simulink model "ADPSE1LEMK"  (R2018b)
settings: Solver=ode1  StartTime=0.0  StopTime=100  FixedStep=1/1000  RelTol=1e-3  AbsTol=1e-3  EnableMultiTasking=on
PostLoadFcn:
  | f_Simulink_figureplace
InitFcn:
  | ADPSE1LEMK_PreSim
values from neighbouring files (symbols this model uses):
  beta = 3    [ADPSE1LEMK_PreSim.m]
  etaa1 = 10    [ADPSE1LEMK_PreSim.m]
  etaa2 = 0.1    [ADPSE1LEMK_PreSim.m]
  etac1 = 1    [ADPSE1LEMK_PreSim.m]
  etac2 = 2    [ADPSE1LEMK_PreSim.m]
  Gamma0 = 100*eye(L)    [ADPSE1LEMK_PreSim.m]
  GammaBar = 100000    [ADPSE1LEMK_PreSim.m]
  GG = [GG;phi_pc*Gc*(R\Gc')*phi_pc']    [ADPSE1LEMK_PreSim.m]
  L = 3    [ADPSE1LEMK_PreSim.m]
  N = length(Xc)^n    [ADPSE1LEMK_PreSim.m]
  PHIPY = [PHIPY;phi_pc*Yc]    [ADPSE1LEMK_PreSim.m]
  Q = [1 0 ; 0 1]    [ADPSE1LEMK_PreSim.m]
  R = 1    [ADPSE1LEMK_PreSim.m]
  v = 0.005    [ADPSE1LEMK_PreSim.m]
  WaH0 = 1*WcH0    [ADPSE1LEMK_PreSim.m]
  WcH0 = 0.2*[1 1 1]'    [ADPSE1LEMK_PreSim.m]
  x0 = [-1;1]    [ADPSE1LEMK_PreSim.m]
  XQX = zeros(N,1)    [ADPSE1LEMK_PreSim.m]
settings Model: Creator=rkamalapurkar  LastModifiedBy=rushik
settings SolverCC: AutoScaleAbsTol=off
settings DataIOCC: SaveFormat=StructureWithTime  SaveOutput=off  SaveTime=off
settings OptimizationCC: ExpressionDepthLimit=2147483647  LifeSpan=inf
settings DebuggingCC: UnderspecifiedInitializationDetection=Classic  MergeDetectMultiDrivingBlocksExec=none  SolverPrmCheckMsg=warning  FcnCallInpInsideContextMsg=warning  StateNameClashWarn=warning  SFUnexpectedBacktrackingDiag=warning  SFNoUnconditionalDefaultTransitionDiag=warning  SFExecutionAtInitializationDiag=none
settings HardwareCC: ProdBitPerPointer=32  ProdBitPerSizeT=32  ProdBitPerPtrDiffT=32  ProdLargestAtomicFloat=None  ProdIntDivRoundTo=Undefined  ProdEndianess=Unspecified  ProdWordSize=32  ProdHWDeviceType=32-bit Generic
settings ModelReferenceCC: PropagateSignalLabelsOutOfModel=off
settings SFSimCC: SimUseLocalCustomCode=off
settings RTWCC: RTWUseLocalCustomCode=off
settings CodeAppCC: StateflowObjectComments=on
settings GRTTargetCC: TargetLangStandard=C89/C90 (ANSI)  GeneratePreprocessorConditionals=Disable all  CombineOutputUpdateFcns=off  GRTInterface=on
settings ConfigComp: CovMetricSettings=dw  CovHtmlReporting=on  CovSaveCumulativeToWorkspaceVar=on  CovSaveSingleToWorkspaceVar=on  CovExternalEMLEnable=off  CovSFcnEnable=off

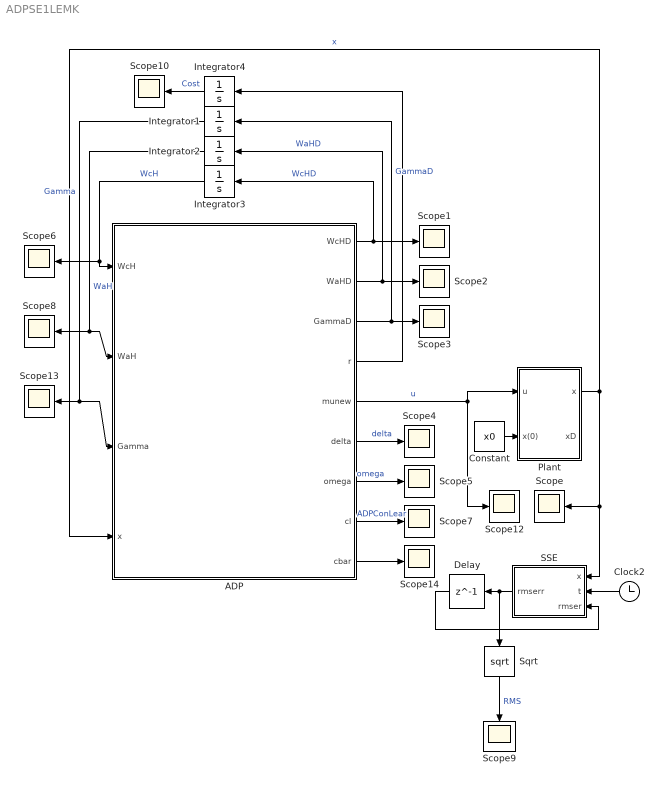
== system ADPSE1LEMK ==
  ADP : MATLAB Function  TreatAsAtomicUnit=on
  Clock2 : Clock
  Constant : Constant  Value=x0
  Delay : Delay  DelayLength=1  InitialCondition=0
  Integrator1 : Integrator  InitialCondition=Gamma0
  Integrator2 : Integrator  InitialCondition=WaH0
  Integrator3 : Integrator  InitialCondition=WcH0
  Integrator4 : Integrator
  Plant : Subsystem
  SSE : MATLAB Function  TreatAsAtomicUnit=on
  Scope{,1..10,12..14} (14 alike) : Scope
  Sqrt : Sqrt  SaturateOnIntegerOverflow=on
  wires:
  ADP/3(GammaD) -> Integrator1/1, Scope3/1  "GammaD"
  ADP/1(WcHD) -> Scope1/1, Integrator3/1  "WcHD"
  Integrator3/1 -> Scope6/1, ADP/1(WcH)  "WcH"
  ADP/2(WaHD) -> Integrator2/1, Scope2/1  "WaHD"
  Integrator2/1 -> ADP/2(WaH), Scope8/1  "WaH"
  ADP/6(delta) -> Scope4/1  "delta"
  ADP/7(omega) -> Scope5/1  "omega"
  Integrator1/1 -> Scope13/1, ADP/3(Gamma)  "Gamma"
  ADP/5(munew) -> Plant/1(u), Scope12/1  "u"
  ADP/8(cl) -> Scope7/1  "ADPConLear"
  Plant/1(x) -> ADP/4(x), SSE/1(x), Scope/1  "x"
  Constant/1 -> Plant/2(x(0))
  ADP/9(cbar) -> Scope14/1
  Clock2/1 -> SSE/2(t)
  SSE/1(rmserr) -> Sqrt/1, Delay/1
  Delay/1 -> SSE/3(rmser)
  Sqrt/1 -> Scope9/1  "RMS"
  ADP/4(r) -> Integrator4/1
  Integrator4/1 -> Scope10/1  "Cost"

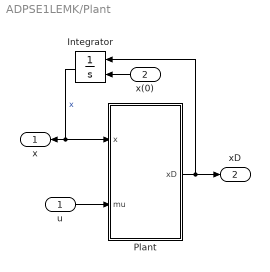
== system ADPSE1LEMK/Plant ==
  u : Inport
  x(0) : Inport  Port=2
  Integrator : Integrator  InitialConditionSource=external  InitialCondition=[1;1;0.0;0.0]
  Plant : MATLAB Function  TreatAsAtomicUnit=on
  x : Outport
  xD : Outport  Port=2
  wires:
  Plant/1(xD) -> Integrator/1, xD/1
  Integrator/1 -> Plant/1(x), x/1  "x"
  u/1 -> Plant/2(mu)
  x(0)/1 -> Integrator/2

== matlab function ADPSE1LEMK/Plant/Plant ==
  data: xD output; x input; mu input
function xD = dynamics(x,mu)
%#codegen
F=[-x(1)+x(2) ;-0.5*x(1)-0.5*x(2)*(1-(cos(2*x(1))+2)^2)];
G=[0; (cos(2*x(1))+2)];
xD = F+G*mu;

== matlab function ADPSE1LEMK/ADP ==
  data: WcH input; WaH input; Gamma input; x input; R parameter; Q parameter; etaa1 parameter; etaa2 parameter; etac1 parameter; etac2 parameter; v parameter; XQX parameter; GG parameter; PHIPY parameter; N parameter; WcHD output; WaHD output; GammaD output; r output; munew output; delta output; omega output; cl output; L parameter; beta parameter; GammaBar parameter; cbar output
function [WcHD,WaHD,GammaD,r,munew,delta,omega,cl,cbar]=...
    control(WcH,WaH,Gamma,x,R,Q,etaa1,etaa2,...
    etac1,etac2,v,XQX,GG,PHIPY,N,L,beta,GammaBar)
%#codegen
thetaS=[-1 1 -0.5 -0.5]'; % True values of SysID Parameters

G = [0 ; (cos(2*x(1))+2)];
Y = [x(1) x(2) 0 0;0 0 x(1) x(2)*(1-(cos(2*x(1))+2)^2)];

phi_p =[2*x(1) 0; x(2) x(1); 0 2*x(2)];

mu=-0.5*(R\G')*phi_p'*WaH;
% pe = sin(2*pi*t) + sin(exp(1)*t) + cos(5*t)^5 ;
munew = mu;

theta = thetaS;
%% Concurrent Learning

GGWaH = reshape(GG*WaH,L,N);
PHIPYtheta = reshape(PHIPY*theta,L,N);
deltac = (PHIPYtheta')*WcH + XQX-(1/2)*(GGWaH'*WcH)+(1/4)*(GGWaH'*WaH);
Omegac = (PHIPYtheta-(1/2)*(GGWaH));
normm=1./(1.+v.*dot(Omegac.',Omegac.'*Gamma.',2));
cbar = real(min(eig(Omegac*diag(normm)*Omegac')));
cl = (-etac2*Gamma*Omegac*diag(normm)*deltac/N);

%% ADP
omega = phi_p*(Y*theta+G*mu);
Gsigma = phi_p*G*(R\G')*phi_p';
r = x'*Q*x + mu'*R*mu;
delta = WcH'*omega + r;
rho = (1+v*omega'*(Gamma)*omega);
WcHD = (-etac1*Gamma*omega*delta/rho+cl);
GammaD = (beta*Gamma-Gamma*(omega*omega'/rho^2)*Gamma)*(norm(Gamma)<=GammaBar);
WaHD = etaa1*(WcH-WaH)...
    -(etaa2*WaH+etac1*Gsigma'*WaH*omega'*WcH/(4*rho))...
    +(etac2*GGWaH*(Omegac*diag(normm))'*WcH/(4*N));

== matlab function ADPSE1LEMK/SSE ==
  data: x input; t input; rmser input; rmserr output
function rmserr = fcn(x,t,rmser)
%#codegen

if t>90
    rmserr = rmser+(1/10000)*(norm(x))^2;
else
    rmserr = 0;
end
